simulink model "moteur_model"  (R2025b)
settings: Solver=VariableStepAuto  StartTime=0.0  StopTime=T  RelTol=1e-3
values from neighbouring files (symbols this model uses):
  A = [-10   1 ... (first row only)    [moteur.m]
  Ad = ssd.A    [moteur.m]
  B = [0 ... (first row only)    [moteur.m]
  Bd = ssd.B    [moteur.m]
  C = [1 0]    [moteur.m]
  d = 10    [moteur.m]
  Ed = A\(expm(A*Ts)-eye(2))*E    [moteur.m]
  F = place(A, B, p_cmd)    [moteur.m]
  Fd = place(Ad, Bd, p_cmd_d)    [moteur.m]
  Fd_aug = place(Ad_aug, Bd_aug, p_cmdi_d)    [moteur.m]
  G = - 1 / (C*inv(A - B*F)* B)    [moteur.m]
  Gd = 1 / (C * ((eye(2) - (Ad - Bd*Fd)) \ Bd))    [moteur.m]
  L = place(A', C', p_obs)'    [moteur.m]
  Ld = place(Ad', C', p_obs_d)'    [moteur.m]
  r = 5    [moteur.m]
  Ts = 0.05    [moteur.m]
undefined symbols (not defined in the file or in its folder): DiscIntNeverNeededParam
settings Model: Creator=victor  LastModifiedBy=victor

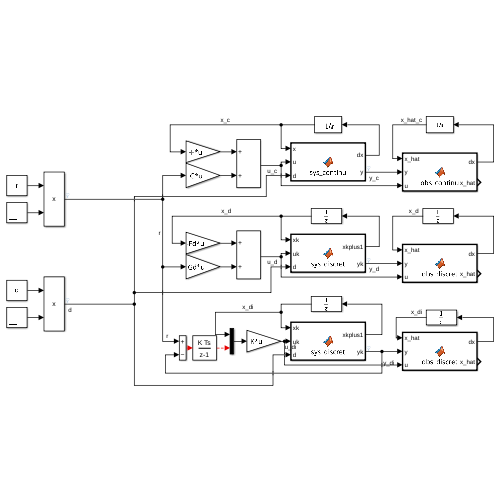
[thumbnail: Simulink's stored preview of the top-level diagram]
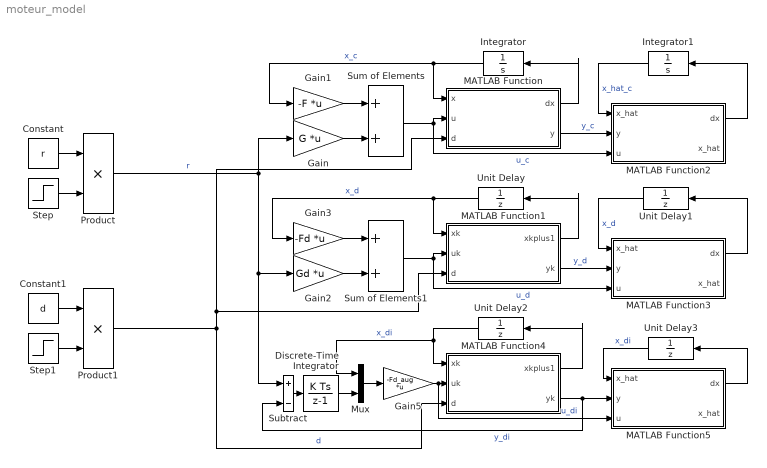
== system moteur_model ==
  Constant : Constant  Value=r
  Constant1 : Constant  Value=d
  Discrete-Time Integrator : DiscreteIntegrator  SampleTime=-1  ICPrevOutput=DiscIntNeverNeededParam  ICPrevScaledInput=DiscIntNeverNeededParam
  Gain : Gain  Gain=G  Multiplication=Matrix(K*u)
  Gain1 : Gain  Gain=-F  Multiplication=Matrix(K*u)
  Gain2 : Gain  Gain=Gd  Multiplication=Matrix(K*u)
  Gain3 : Gain  Gain=-Fd  Multiplication=Matrix(K*u)
  Gain5 : Gain  Gain=-Fd_aug  Multiplication=Matrix(K*u)
  Integrator : Integrator
  Integrator1 : Integrator
  MATLAB Function : MATLAB Function  TreatAsAtomicUnit=on
  MATLAB Function1 : MATLAB Function  TreatAsAtomicUnit=on  SystemSampleTime=Ts
  MATLAB Function2 : MATLAB Function  TreatAsAtomicUnit=on
  MATLAB Function3 : MATLAB Function  TreatAsAtomicUnit=on  SystemSampleTime=Ts
  MATLAB Function4 : MATLAB Function  TreatAsAtomicUnit=on  SystemSampleTime=Ts
  MATLAB Function5 : MATLAB Function  TreatAsAtomicUnit=on  SystemSampleTime=Ts
  Mux : Mux  Inputs=[2 1]
  Product : Product
  Product1 : Product
  Step : Step  SampleTime=0
  Step1 : Step  Time=3  SampleTime=0
  Subtract : Sum  Inputs=+-
  Sum of Elements : Sum
  Sum of Elements1 : Sum
  Unit Delay{,1..3} (4 alike) : UnitDelay  SampleTime=-1  HasFrameUpgradeWarning=on
  wires:
  Constant/1 -> Product/1
  Step/1 -> Product/2
  Sum of Elements/1 -> MATLAB Function2/3(u), MATLAB Function/2(u)  "u_c"
  Product/1 -> Gain/1, Subtract/1, Gain2/1  "r"
  Gain2/1 -> Sum of Elements1/2
  Sum of Elements1/1 -> MATLAB Function3/3(u), MATLAB Function1/2(uk)  "u_d"
  Integrator/1 -> MATLAB Function/1(x), Gain1/1  "x_c"
  MATLAB Function/1(dx) -> Integrator/1
  Gain1/1 -> Sum of Elements/1
  Gain/1 -> Sum of Elements/2
  Gain3/1 -> Sum of Elements1/1
  MATLAB Function1/1(xkplus1) -> Unit Delay/1
  Unit Delay/1 -> MATLAB Function1/1(xk), Gain3/1  "x_d"
  MATLAB Function/2(y) -> MATLAB Function2/2(y)  "y_c"
  Integrator1/1 -> MATLAB Function2/1("x_hat ")  "x_hat_c"
  MATLAB Function2/1(dx) -> Integrator1/1
  MATLAB Function1/2(yk) -> MATLAB Function3/2(y)  "y_d"
  Unit Delay1/1 -> MATLAB Function3/1("x_hat ")  "x_d"
  MATLAB Function3/1(dx) -> Unit Delay1/1
  Unit Delay2/1 -> Mux/1, MATLAB Function4/1(xk)  "x_di"
  MATLAB Function4/1(xkplus1) -> Unit Delay2/1
  MATLAB Function4/2(yk) -> MATLAB Function5/2(y), Subtract/2  "y_di"
  Subtract/1 -> Discrete-Time Integrator/1
  Mux/1 -> Gain5/1
  Step1/1 -> Product1/2
  Constant1/1 -> Product1/1
  Product1/1 -> MATLAB Function4/3(d), MATLAB Function/3(d), MATLAB Function1/3(d)  "d"
  Gain5/1 -> MATLAB Function5/3(u), MATLAB Function4/2(uk)  "u_di"
  Discrete-Time Integrator/1 -> Mux/2
  Unit Delay3/1 -> MATLAB Function5/1("x_hat ")  "x_di"
  MATLAB Function5/1(dx) -> Unit Delay3/1

== matlab function moteur_model/MATLAB Function1 ==
  data: xk input; xkplus1 output; uk input; d input; yk output; Ad parameter; Bd parameter; C parameter; Ed parameter
function [xkplus1, yk] = sys_discret(xk, uk, d, Ad, Bd, C, Ed)
xkplus1 = zeros(2, 1); 
yk = 0;
xkplus1 = Ad*xk + Bd*uk +Ed*d;
yk = C*xk;

== matlab function moteur_model/MATLAB Function ==
  data: x input; dx output; u input; d input; y output; A parameter; B parameter; C parameter; E parameter
function [dx, y] = sys_continu(x, u, d, A, B, C, E)
dx = zeros(2, 1); 
y = 0;
dx = A*x + B*u + E*d;
y = C*x;

== matlab function moteur_model/MATLAB Function2 ==
  data: x_hat input; y input; dx output; u input; A parameter; B parameter; C parameter; L parameter; x_hat output
function [dx, x_hat]  = obs_continu(x_hat, y, u, A, B, C, L)
dx = zeros(2, 1);
y_hat = C*x_hat;
dx = A*x_hat + B*u + L*(y-y_hat);

== matlab function moteur_model/MATLAB Function3 ==
  data: x_hat input; y input; dx output; u input; Ad parameter; Bd parameter; C parameter; Ld parameter; x_hat output
function [dx, x_hat]  = obs_discret(x_hat, y, u, Ad, Bd, C, Ld)
dx = zeros(2, 1);
y_hat = C*x_hat;
dx = Ad*x_hat + Bd*u + Ld*(y-y_hat);

== matlab function moteur_model/MATLAB Function4 ==
  data: xk input; xkplus1 output; uk input; d input; yk output; Ad parameter; Bd parameter; C parameter; Ed parameter
function [xkplus1, yk] = sys_discret(xk, uk, d, Ad, Bd, C, Ed)
xkplus1 = zeros(2, 1); 
yk = 0;
xkplus1 = Ad*xk + Bd*uk +Ed*d;
yk = C*xk;

== matlab function moteur_model/MATLAB Function5 ==
  data: x_hat input; y input; dx output; u input; Ad parameter; Bd parameter; C parameter; Ld parameter; x_hat output
function [dx, x_hat]  = obs_discret(x_hat, y, u, Ad, Bd, C, Ld)
dx = zeros(2, 1);
y_hat = C*x_hat;
dx = Ad*x_hat + Bd*u + Ld*(y-y_hat);
